simulink model "Simulink_Model__Carl_Johan_Larsson_Gustaf_Rydholm"  (R2014a)
settings: Solver=ode45  StartTime=0.0  StopTime=10.0  RelTol=1e-3
undefined symbols (not defined in the file or in its folder): Fs
libraries: dspsnks4 x1, dspsrcs4 x1
settings Model: Creator=Carl-Johan  LastModifiedBy=Carl-Johan

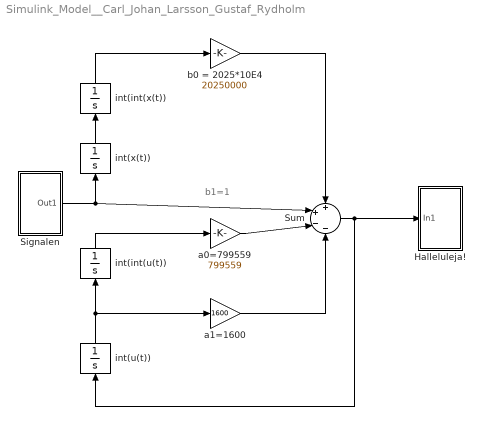
== system Simulink_Model__Carl_Johan_Larsson_Gustaf_Rydholm ==
  note: b1=1
  Halleluleja! : Subsystem  mask{Fs=8192, gain=0.06}
      mask prompts: Fs "Samplingsfrekvens"; gain "Amplitudskalning"
      mask Display:
      | icon = dspdialog.ToAudioDevice.maskInit();
      | patch(icon.x1, icon.y1,[1 1 1]*.5);
      | patch(icon.x2, icon.y2);
      | plot(icon.x, icon.y);
      | plot(icon.x1, icon.y1);
  Signalen : Subsystem  mask{Birthday=900821}
      mask prompts: Birthday "Födelsedag (YYDDMM)"
      mask init:
      | if Birthday < 1e5 || Birthday >=1e6
      |     warndlg('Skriv födelsedagen på formatet YYMMDD')
      | end
      | 
      | YY=floor(Birthday/1e4);
      | MM=floor(rem(Birthday,1e4)/100);
      | DD=rem(Birthday,100);
      | 
      | w0=50*YY;
      | %p=25*YY+10*DD;
      | b1=200*MM;
      | b0=1e4*MM^2-DD^2;
      | 
      | load handel
      mask Display: port_label('output',1,'x(t)')
  Sum : Sum  Inputs=++--
  a0=799559 : Gain  Gain=799559
  a1=1600 : Gain  Gain=1600
  b0 = 2025*10E4 : Gain  Gain=20250000
  int(int(u(t)) : Integrator
  int(int(x(t)) : Integrator
  int(u(t)) : Integrator
  int(x(t)) : Integrator
  wires:
  Signalen/1(Out1) -> int(x(t))/1, Sum/2
  int(x(t))/1 -> int(int(x(t))/1
  int(int(x(t))/1 -> b0 = 2025*10E4/1
  b0 = 2025*10E4/1 -> Sum/1
  Sum/1 -> Halleluleja!/1(In1), int(u(t))/1
  int(u(t))/1 -> int(int(u(t))/1, a1=1600/1
  int(int(u(t))/1 -> a0=799559/1
  a1=1600/1 -> Sum/4
  a0=799559/1 -> Sum/3

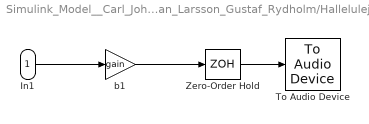
== system Simulink_Model__Carl_Johan_Larsson_Gustaf_Rydholm/Halleluleja! ==
  In1 : Inport
  To Audio Device : dspsnks4/To Audio Device  deviceName=Default  inheritSampleRate=on  sampleRate=44100  deviceDatatype=Determine from input data type  autoBufferSize=on  bufferSize=4096  queueDuration=1.0  defaultOutputChannelMapping=on  outputChannelMapping=1
  Zero-Order Hold : ZeroOrderHold  SampleTime=1/Fs
  b1 : Gain  Gain=gain
  wires:
  Zero-Order Hold/1 -> To Audio Device/1
  In1/1 -> b1/1
  b1/1 -> Zero-Order Hold/1

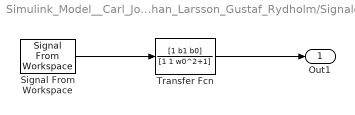
== system Simulink_Model__Carl_Johan_Larsson_Gustaf_Rydholm/Signalen ==
  Signal From Workspace : dspsrcs4/Signal From Workspace  X=y  Ts=1/Fs  nsamps=1  OutputAfterFinalValue=Setting to zero  ignoreOrWarnInputAndFrameLengths=off
  Transfer Fcn : TransferFcn  Numerator=[1 b1 b0]  Denominator=[1 1 w0^2+1]
  Out1 : Outport
  wires:
  Signal From Workspace/1 -> Transfer Fcn/1
  Transfer Fcn/1 -> Out1/1
